simulink model "sampling"  (R2023b)
settings: Solver=VariableStepAuto  StartTime=0.0  StopTime=10.0  RelTol=1e-3
settings Model: Creator=ASUS  LastModifiedBy=ASUS

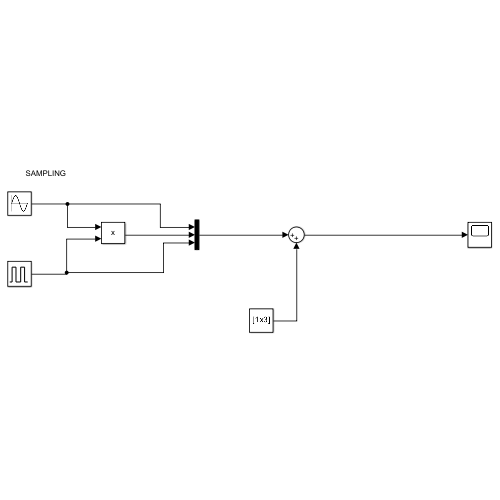
[thumbnail: Simulink's stored preview of the top-level diagram]
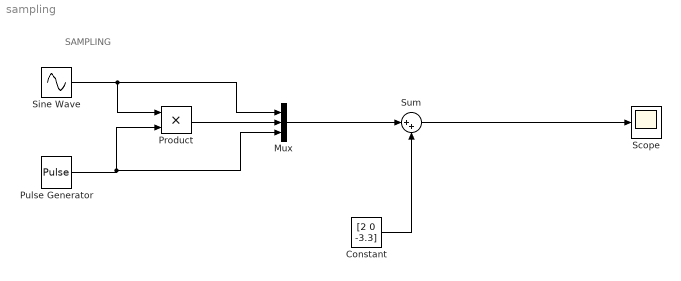
== system sampling ==
  note: SAMPLING
  Constant : Constant  Value=[2 0 -3.3]
  Mux : Mux  Inputs=3
  Product : Product
  Pulse Generator : DiscretePulseGenerator  PulseType=Time based  Amplitude=1.5  Period=0.025  PulseWidth=50
  Scope : Scope
  Sine Wave : Sin  Frequency=2*pi  SampleTime=0
  Sum : Sum  Inputs=|++
  wires:
  Product/1 -> Mux/2
  Pulse Generator/1 -> Mux/3, Product/2
  Sine Wave/1 -> Mux/1, Product/1
  Constant/1 -> Sum/2
  Mux/1 -> Sum/1
  Sum/1 -> Scope/1
